simulink model "Chassis"  (R2015a)
settings: Solver=ode45  StartTime=0.0  StopTime=10.0  RelTol=1e-3
settings Model: Creator=laragoxhaj  LastModifiedBy=laragoxhaj

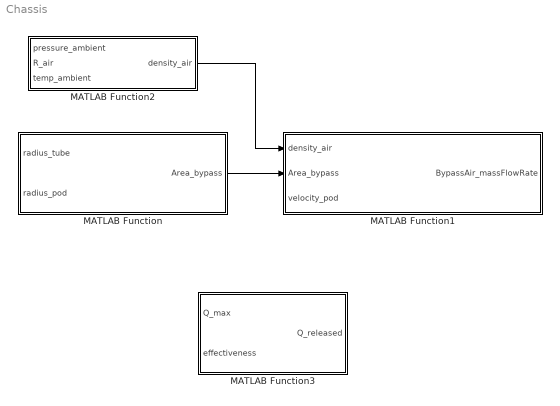
== system Chassis ==
  MATLAB Function : MATLAB Function  TreatAsAtomicUnit=on
  MATLAB Function1 : MATLAB Function  TreatAsAtomicUnit=on
  MATLAB Function2 : MATLAB Function  TreatAsAtomicUnit=on
  MATLAB Function3 : MATLAB Function  TreatAsAtomicUnit=on
  wires:
  MATLAB Function/1(Area_bypass) -> MATLAB Function1/2(Area_bypass)
  MATLAB Function2/1(density_air) -> MATLAB Function1/1(density_air)

== matlab function Chassis/MATLAB Function1 ==
  data: density_air input; Area_bypass input; velocity_pod input; BypassAir_massFlowRate output
% kg/s^2
function BypassAir_massFlowRate = fcn(density_air, Area_bypass, velocity_pod)
BypassAir_massFlowRate = density_air * Area_bypass * velocity_pod;

% Max flow rate occurs when velocity reaches Mach 1

== matlab function Chassis/MATLAB Function ==
  data: radius_tube input; Area_bypass output; radius_pod input
% m^2
function Area_bypass = fcn(radius_tube, radius_pod)
Area_bypass = pi*(radius_tube^2 - radius_pod^2);

== matlab function Chassis/MATLAB Function2 ==
  data: pressure_ambient input; R_air input; temp_ambient input; density_air output
% kg/m^3
function density_air = fcn(pressure_ambient, R_air, temp_ambient)
density_air = pressuree_ambient / (R_air * temp_ambient);

== matlab function Chassis/MATLAB Function3 ==
  data: Q_max input; Q_released output; effectiveness input
% J
function Q_released = fcn(Q_max, effectiveness)
Q_released = Q_max * effectiveness;
